simulink model "HostOfSeal"  (R2025a)
settings: Solver=FixedStepDiscrete  StartTime=0.0  StopTime=30  FixedStep=0.025  RelTol=1e-3
model workspace (MATLAB code in the model file + MAT data in the model file):
  | cmdLim = Simulink.Parameter;
  | cmdLim.Value = 15;
  | cmdLim.Description = 'Limit for controlling the maximum surface command angle.';
  | cmdLim.Min = 0;
  | cmdLim.Max = 90;
  | cmdLim.DocUnits = 'deg';
  | 
  | dispGain = Simulink.Parameter;
  | dispGain.Value = 0.75;
  | dispGain.Description = 'Gain applied to the displacement error.';
  | dispGain.Min = 0;
  | dispGain.Max = [];
  | dispGain.DocUnits = 'deg/sec/deg';
  | 
  | dispLim = Simulink.Parameter;
  | dispLim.Value = 30;
  | dispLim.Description = 'Limit for controlling the maximum commanded angle.';
  | dispLim.Min = 0;
  | dispLim.Max = 180;
  | dispLim.DocUnits = 'deg';
  | 
  | intGain = Simulink.Parameter;
  | intGain.Value = 0.5;
  | intGain.Description = 'Gain applied to the integral error.';
  | intGain.Min = 0;
  | intGain.Max = [];
  | intGain.DocUnits = 'deg/sec/deg/sec';
  | 
  | intLim = Simulink.Parameter;
  | intLim.Value = 5;
  | intLim.Description = 'Limit for controlling the maximum commanded angle.';
  | intLim.Min = 0;
  | intLim.Max = 90;
  | intLim.DocUnits = 'deg';
  | 
  | rateGain = Simulink.Parameter;
  | rateGain.Value = 2;
  | rateGain.Description = 'Gain applied to the rate error.';
  | rateGain.Min = 0;
  | rateGain.Max = [];
  | rateGain.DocUnits = 'deg/deg/sec';
  | 
  | rateLim = Simulink.Parameter;
  | rateLim.Value = 6;
  | rateLim.Description = 'Limit for controlling the maximum commanded angle.';
  | rateLim.Min = 0;
  | rateLim.Max = 180;
  | rateLim.DocUnits = 'deg/sec';
  | 
  | hdgGain = Simulink.Parameter;
  | hdgGain.Value = 0.015;
values from neighbouring files (symbols this model uses):
  DriveTs = 100e-6    (= 0.0001)    [simpars.m]
  Jm = 1    [simpars.m]
  KEp = Kt * sqrt(2) / 1.5    [simpars.m]
  Kt = 1    [simpars.m]
  Lm = 1e-3    (= 0.001)    [simpars.m]
  PolePairs = 5    [simpars.m]
  Rm = 1    [simpars.m]
  Vdc = 24    [simpars.m]
undefined symbols (not defined in the file or in its folder): CurrentCommand, DcBusVoltage, EncoderMain, EncoderMainSpeed, Iq, KiSpeed, Kp, KpSpeed, PositionCommand, SpeedCommand, SystemTime
libraries: simulink x1
(part 2 of 2)

== matlab function HostOfSeal/Gft Servo Drive with SEAL/SEAL/100 usec Periodic profiler/MATLAB Function ==
  data: y output double size=[3,1]; G_PosProfilerState data_store_memory; G_PosProfilerData data_store_memory; G_SetupReportBuf data_store_memory
function y  = fcn

global G_PosProfilerState
global G_PosProfilerData
global G_SetupReportBuf

Ts = double( G_PosProfilerData.Ts) ; 
% Copy state for use 

y = zeros(3,1) ; 
if ( G_PosProfilerData.ProfileDataOk == 0 )
    speed =  max( abs(G_PosProfilerState.Speed)-Ts*G_SetupReportBuf.AbsoluteAccelerationLimit , 0 ) * sign(G_PosProfilerState.Speed); 
    pos    = G_PosProfilerState.Position + ( speed + G_PosProfilerState.Speed ) * Ts* 0.5  ;  
    NewFiltState4 = double(pos) ; 
    NewFiltState3 = double(pos) ; 
    NewFiltState2 = double(pos) ; 
    NewFiltState1 = double(pos) ; 
else  
    % Advance profiler 
    Delta = G_PosProfilerData.PositionTarget - G_PosProfilerState.Position - G_PosProfilerState.Speed * Ts * 0.5  ; 
    Direction = 1 ; 
    if ( Delta < 0  )
        Direction = -1 ; 
        Delta = -Delta ;
        speed  = -G_PosProfilerState.Speed ; 
    else
        speed  = G_PosProfilerState.Speed ; 
    end 
        
    desiredSpeed = sqrt(Delta * 2 * G_PosProfilerData.ProfileDeceleration ) ; 
    if ( speed < desiredSpeed  ) 
        speed = min ([speed +Ts * G_PosProfilerData.ProfileDeceleration , G_PosProfilerData.ProfileSpeed  , desiredSpeed] ) ; 
    else
        speed = max(desiredSpeed , speed - Ts * G_PosProfilerData.ProfileDeceleration * 1.02   ) ;  
    end
    speed = speed * Direction ; 

    % tf(2 ,conv([1,2],[1,1.71,1]) )
    pos    = G_PosProfilerState.Position + ( speed +  G_PosProfilerState.Speed ) * Ts* 0.5  ;  
    NewFiltState4 = G_PosProfilerState.FiltState(3) ; 
    NewFiltState3 = G_PosProfilerState.FiltState(2) ; 
    NewFiltState2 = G_PosProfilerState.FiltState(1) ;
    NewFiltState1 = -(G_PosProfilerState.FiltState(1) * G_PosProfilerData.ProfileFilterDen(2) + ...
        G_PosProfilerState.FiltState(2) * G_PosProfilerData.ProfileFilterDen(3) + ...
        G_PosProfilerState.FiltState(3) * G_PosProfilerData.ProfileFilterDen(4)) + double(pos) * G_PosProfilerData.ProfileFilterNum ; 

end
G_PosProfilerState.Position =  double(pos)   ; 
G_PosProfilerState.Speed    =  double(speed) ; 
y = [NewFiltState1 ; (NewFiltState1-G_PosProfilerState.FiltState(1))/ max(Ts,1e-5); 0 ] ;  
G_PosProfilerState.FiltState = [NewFiltState1;NewFiltState2;NewFiltState3;NewFiltState4] ;

end

== matlab function HostOfSeal/Gft Servo Drive with SEAL/SEAL/Idle process UART interpreter/UART message response ==
  data: G_pUartCyclicBuf_in data_store_memory; G_pUartCyclicBuf_out data_store_memory; G_MicroInterp data_store_memory
function UARTHandler()

%global   
global G_MicroInterp      
global G_pUartCyclicBuf_in

for cnt = 1:10 
% The CAN queues count like C (zero based), yet the code here is matlab (1
% based) so we have to increment the counters to be valid Matlab indices
    if (G_pUartCyclicBuf_in.PutCounter == G_pUartCyclicBuf_in.FetchCounter ) 
        return ; 
    end

    nmsgGet     = bitand( G_pUartCyclicBuf_in.FetchCounter, 255) ; 
    nextfetch   = bitand( nmsgGet + 1, 255 ); 
    nextmsg     = G_pUartCyclicBuf_in.UARTQueue(nmsgGet + 1 ) ;
    G_pUartCyclicBuf_in.FetchCounter = nextfetch ; 

    if G_pUartCyclicBuf_in.UartError 
        G_pUartCyclicBuf_in.UartError = uint16(0) ; 
        G_MicroInterp.InterpretError = uint16(3) ; 
        continue ; 
    end

    StringFormatter(nextmsg) ; 
    if ( G_MicroInterp.NewString )
        StringMicroSplitter() ;  
        if G_MicroInterp.InterpretError== uint16(0) 
            MicroInterpret() ; 
            FormatInterpreterResponse() ;
            SendTxResponse();
        end
    end
end
end

function FormatInterpreterResponse() 
    global G_MicroInterp 
    if ( G_MicroInterp.InterpretError) 
        
            
        G_MicroInterp.TempString(1) = 'E' ; 
        G_MicroInterp.TempString(2) = 'R' ; 
        G_MicroInterp.TempString(3) = 'R' ; 
        G_MicroInterp.TempString(4) = 'O' ; 
        G_MicroInterp.TempString(5) = 'R' ; 
        G_MicroInterp.TempString(6) = ':' ; 
        G_MicroInterp.cnt = uint16(6) ; 
        errnum = G_MicroInterp.InterpretError ; 
        while ( errnum )
            G_MicroInterp.cnt = G_MicroInterp.cnt + uint16(1) ;
            nextdigit = uint16(mod( errnum , 10 )) ; 
            G_MicroInterp.TempString(G_MicroInterp.cnt) = nextdigit + uint16('0') ; 
            errnum = errnum - nextdigit ;
        end
    end

    if ( G_MicroInterp.IsGetFunc) 
        n = fix(log10(G_MicroInterp.Argument)) ; 
        SciExp = int16(0) ; 
        SciNotation = 0 ; 
        argout = G_MicroInterp.Argument  ;
        if n > 8 || n < -8   
            nafterPeriod = 8 - n  ; 
        else
            nafterPeriod = 6   ; 
            SciNotation  = 1   ; 
            SciExp = int16(n) ; 
            argout = argout * 10^(-n) ; 
            %n = 1 ; 
        end

        m = fix(argout) ; 
        while ( m )
            G_MicroInterp.cnt = G_MicroInterp.cnt + 1 ;
            nextdigit = uint16(mod( m , 10 )) ; 
            G_MicroInterp.TempString(G_MicroInterp.cnt) = nextdigit + uint16('0') ; 
            m = m - double(nextdigit) ;
        end
        if nafterPeriod > 0 
            G_MicroInterp.cnt = G_MicroInterp.cnt + 1 ;
            G_MicroInterp.TempString(G_MicroInterp.cnt) = '.' ; 
            m = fix( (argout-m) * 10^(nafterPeriod)) ; 
            while ( m )
                G_MicroInterp.cnt = G_MicroInterp.cnt + 1 ;
                nextdigit = uint16(mod( m , 10 )) ; 
                G_MicroInterp.TempString(G_MicroInterp.cnt) = nextdigit + uint16('0') ; 
                m = m - double(nextdigit) ;
            end                
        end
        if SciNotation && SciExp 
            G_MicroInterp.cnt = G_MicroInterp.cnt + 1 ;
            G_MicroInterp.TempString(G_MicroInterp.cnt) = 'E' ; 
            if ( SciExp < 0 )

                G_MicroInterp.cnt = G_MicroInterp.cnt + 1 ;
                G_MicroInterp.TempString(G_MicroInterp.cnt) = '-' ; 
                SciExp = -SciExp ; 
            end
            while ( SciExp )
                G_MicroInterp.cnt = G_MicroInterp.cnt + 1 ;
                nextdigit = uint16(mod( SciExp , 10 )) ; 
                G_MicroInterp.TempString(G_MicroInterp.cnt) = nextdigit + uint16('0') ; 
                SciExp = SciExp - int16(nextdigit) ;
            end                
        end

    end
end


function SendTxResponse()
% Transmit text to a cyclic buffer
    % Return interpreter response 
    global G_pUartCyclicBuf_out  
    global G_MicroInterp      
    for txcnt = 1 : G_MicroInterp.cnt
        nput    = bitand( G_pUartCyclicBuf_out.PutCounter  , 255)  ; 
        nextput = bitand( nput + 1 , 255)  ;  
        if ( nextput == G_pUartCyclicBuf_out.FetchCounter) 
            break ; % Output queue is full 
        end 
        G_pUartCyclicBuf_out.UARTQueue( nput+1) = G_MicroInterp.TempString(txcnt) ; 
    
        % Update TX counter
        G_pUartCyclicBuf_out.PutCounter  = nextput ;
    end
end

function MicroInterpret() 
    global G_MicroInterp      
    switch (G_MicroInterp.MnemonicIndex) 
        case 390 % PA 
            if ( G_MicroInterp.IsGetFunc )
                G_MicroInterp.Argument = GetPositionTarget() ; 
            else
                G_MicroInterp.InterpretError = SetPositionTarget(G_MicroInterp.Argument) ;  
            end
        otherwise
             G_MicroInterp.InterpretError = uint16(22); 

    end
end

function  StringFormatter(c) 

    arguments (Input)
        c uint16 
    end

    global G_MicroInterp      
    
    if ( c == ';' )
        G_MicroInterp.NewString = G_MicroInterp.cnt ; 
        return    ; 
    end
    if G_MicroInterp.NewString 
        G_MicroInterp.cnt = uint16(0) ; 
        G_MicroInterp.InterpretError = uint16(0); 
    end 

    if G_MicroInterp.InterpretError  
        return 
    end

    if ( c <= 'z' && c >= 'a')
        c = c + uint16('A') - uint16('a')   ; 
    end

    if ( c >= 9 && c <= 13) || (c == 32) || (c=='+')
        return ; %  Whitespace - ignore 
    end

    if ( G_MicroInterp.cnt >= 64 )
        G_MicroInterp.InterpretError = uint16(2) ; 
    end

    if ( c <= 'Z' && c >= 'A') || ( c <= '9' && c >= '0') || (c=='-') || (c=='=')
          G_MicroInterp.TempString(G_MicroInterp.cnt+1)  ; 
          G_MicroInterp.cnt = G_MicroInterp.cnt+1 ;
    else
        G_MicroInterp.InterpretError =  uint16(1) ; 
    end

end


function StringMicroSplitter() 
    global G_MicroInterp      
    G_MicroInterp.NewString = uint16(0) ;
    if (G_MicroInterp.cnt < 2 ) 
        return ; 
    end
    if  (G_MicroInterp.TempString(1) < 'A') || (G_MicroInterp.TempString(1) > 'Z') || ...
            (G_MicroInterp.TempString(2) < 'A') || (G_MicroInterp.TempString(2) > 'Z')  
        G_MicroInterp.InterpretError = uint16(10);  
        return ; 
    end
    G_MicroInterp.IsGetFunc  = uint16(1) ; 
    G_MicroInterp.ArrayIndex = uint16(1) ; 
    
    G_MicroInterp.MnemonicIndex = G_MicroInterp.TempString(1) * 26 + G_MicroInterp.TempString(2)  ; 
    
    % Case of scalar GET mnemonic
    if (G_MicroInterp.cnt <= 2 ) 
        return ; 
    end
    
    start = uint16(3) ; 
    if ( G_MicroInterp.TempString(3) =='[')
        gotArrayIndex = uint16(0) ; 
        G_MicroInterp.ArrayIndex = uint16(0) ; 
        for cnt = uint16(4):G_MicroInterp.cnt
            if ( G_MicroInterp.TempString(cnt) == ']')
                if ( G_MicroInterp.ArrayIndex  == 0 ) 
                    G_MicroInterp.InterpretError = uint16(11);  
                    return ; 
                end
                start = cnt + uint16(1) ; 
                gotArrayIndex = uint16(1) ; 
            else
                c = bitand(G_MicroInterp.TempString(cnt), 255 ) ; 
                if ( c < '0' || c > '9')
                    G_MicroInterp.InterpretError =  uint16(12)   ;  
                    return ; 
                end
                G_MicroInterp.ArrayIndex = bitand(G_MicroInterp.ArrayIndex ,31) * 10 + c - uint16('0') ; 
            end
        end
        if ( gotArrayIndex == 0 )
            G_MicroInterp.InterpretError = uint16(14)   ; 
            return ; 
        end
    end

    % Case of vector GET mnemonic
    if (G_MicroInterp.cnt < start ) 
        return ; 
    end
    
    if ~( G_MicroInterp.TempString(start) == '=')
        G_MicroInterp.InterpretError = uint16(15)  ;  
        return ; 
    end
    
    start = start + uint16(1) ;
    Mantissa = 0  ; 
    Exp = uint16(0) ; 
    sgnMant = int16(1) ; 
    sgnExp = int16(1) ; 
    isExp = uint16(0) ; 
    if (G_MicroInterp.cnt < start ) 
        G_MicroInterp.InterpretError = uint16(16)  ;  
        return ; 
    end
    if (G_MicroInterp.TempString(start) == '-')
        sgnMant = int16(-1) ; 
        start = start + uint16(1) ; 
        if (G_MicroInterp.cnt < start ) 
            G_MicroInterp.InterpretError = uint16(17)  ;  
            return ; 
        end
    end

    cnt = start ; 
    WasPeriod = uint16(0); 
    PeriodPos = uint16(0) ; 
    while ( cnt <= G_MicroInterp.cnt) 
        c = bitand(G_MicroInterp.TempString(cnt),255) ;  
        if ( isExp == 0 )
            if ( c >= '0' && c <= '9')
                Mantissa = Mantissa * 10 + double(c)  ; 
                cnt = cnt + uint16(1) ;
                if ( WasPeriod) 
                    PeriodPos = PeriodPos + uint16(1) ;
                end
            else
                if ( c == '.')
                    WasPeriod = uint16(1) ; 
                else
                    if ( c == 'E' )
                        cnt = cnt+ 1 ; 
                        isExp = uint16(1) ;
                        if cnt > G_MicroInterp.cnt
                            G_MicroInterp.InterpretError = uint16(19)  ;  
                            return ; 
                        end
                        if (G_MicroInterp.TempString(cnt) == '-' )
                            sgnExp = int16(-1) ; 
                            cnt = cnt+ uint16(1) ;
                            if cnt > G_MicroInterp.cnt
                                G_MicroInterp.InterpretError = uint16(20)  ;  
                                return ; 
                            end
                        end
                    else
                        G_MicroInterp.InterpretError = uint16(18)  ;  
                        return ; 
                    end
                end
            end
        else
            if ( c >= '0' && c <= '9')
                Exp = bitand(Exp,511) * 10 + c  ; 
                cnt = cnt + 1 ;
            else
                G_MicroInterp.InterpretError = uint16(21)  ;  
                return ;                 
            end
        end
        
    end
    if WasPeriod  
         Mantissa = Mantissa / double(10^single(PeriodPos)) ; 
    end
    G_MicroInterp.Argument = Mantissa * double(sgnMant) ; 
    if isExp
        G_MicroInterp.Argument = G_MicroInterp.Argument * double(10^(single(sgnExp)*single(Exp)) ) ; 
    end

end


function value = GetPositionTarget() 
value = 0 ; 
end

function errcode = SetPositionTarget(pa) 
errcode = uint16(0) ; 
end



% celems(1) = SetBusElement('PutCounter','uint16',"The place in the UARTQueue where the next message is to be put" ) ; 
% celems(2) = SetBusElement('FetchCounter','uint16',"The location in the UARTQueue of the next message to read" ) ; 
% celems(3) = SetBusElement('CANError','uint16',"CAN error" ) ; 
% celems(4) = SetBusElement('UARTQueue','uint32',"Software Queue for incoming UART characters" ,[64,2]) ; 
% celems(5) = SetBusElement('TxFetchCounter','uint16',"The location in the UARTQueue of the next message to transmit" ) ; 
% celems(6) = SetBusElement('CANID','uint32',"Can ID, 11 or 29bit" ,[64,1]) ; 
% celems(7) = SetBusElement('DLenAndAttrib','uint16',"Data length and attributes" ,[64,1]) ;

== matlab function HostOfSeal/Gft Servo Drive with SEAL/SEAL/Drive configuration/MATLAB Function ==
function SealSetup() 

global G_UserInfo

% Object Initialization code 
 SetObject2Drive( uint16(hex2dec('60f0')), uint16(1)  , single(150000) ,VarDataTypes.T_uint32) ; 

% Get object from file 
% G_UserInfo.junk1 = single( GetObjectFromDrive( uint16(hex2dec('60f0')), uint16(1) , VarDataTypes.T_uint32) ) ; 

end


function retCode = SetObject2Drive( Index, subIndex  ,value  , datatype ) 
    retCode = int32(0); 
    coder.ceval('SetObject2Drive', uint16(Index), uint16(subIndex), double(value) , uint16(datatype) ,coder.ref(retCode));
end

function [value,retCode] = GetObjectFromDrive( Index, subIndex , datatype) 
    retCode = int32(0); 
    value   = double(0) ; 
    coder.ceval('GetObjectFromDrive', uint16(Index), uint16(subIndex), uint16(datatype) , coder.ref(value), coder.ref(retCode));
end

== matlab function HostOfSeal/Gft Servo Drive with SEAL/SEAL/Add char to UART/Accept character ==
  data: u input; G_pUartCyclicBuf_in data_store_memory
function ReceiveUartChar(u)

global G_pUartCyclicBuf_in

next = uint16(bitand(G_pUartCyclicBuf_in.PutCounter,255)+ 1) ; 
if ( next == G_pUartCyclicBuf_in.FetchCounter )
    G_pUartCyclicBuf_in.UartError = uint16(1) ; 
    return ; 
end
G_pUartCyclicBuf_in.UARTQueue(G_pUartCyclicBuf_in.PutCounter)  = u ; 
G_pUartCyclicBuf_in.PutCounter = next ;

== matlab function HostOfSeal/Gft Servo Drive with SEAL/SEAL/Copy UART buffer/Get From UART FIFO ==
  data: y output; G_pUartCyclicBuf_out data_store_memory
function y = GetFromUartFifo
global G_pUartCyclicBuf_out 
y = G_pUartCyclicBuf_out ; 
nchars = mod( y.PutCounter - y.FetchCounter, 256 ) ; 
if ( y.PutCounter >= y.FetchCounter)
    y.UARTQueue(1:nchars) = y.UARTQueue(y.FetchCounter:y.FetchCounter+nchars-1) ; 
else
    nrem = 256 - y.FetchCounter + 1  ; 
    y.UARTQueue(1:nrem) = y.UARTQueue(y.FetchCounter:256) ;   
    if ( y.PutCounter > 1 ) 
        y.UARTQueue(nrem+1:nchars)  = y.UARTQueue(1:y.PutCounter-1) ;     
    end
end
y.PutCounter = mod( nchars + 1 , 256) ; 
y.FetchCounter = 1 ; 


% y = uint16([0;0]) ; 
% nchars = mod( G_pUartCyclicBuf_out.PutCounter - G_pUartCyclicBuf_out.FetchCounter, 256 ) ; 
% nextchar = 0 ; 
% if nchars ~= 0 
%     next = uint16(bitand ( G_pUartCyclicBuf_out.FetchCounter, 255) + 1) ; 
%     nextchar = G_pUartCyclicBuf_out.UARTQueue(next) ; 
%     G_pUartCyclicBuf_out.FetchCounter = next ;  
% end
% y(1) = uint16(nextchar) ; 
% y(2) = uint16(nchars) ;

== matlab function HostOfSeal/Gft Servo Drive with SEAL/SEAL/Get CAN Msg to transmit/MATLAB Function ==
  data: y output Bus: CANMessage_T size=1; G_pCANCyclicBuf_out data_store_memory; data input
function y = CanOutTx( data)

global G_pCANCyclicBuf_out 

y = data ; 
if ~(G_pCANCyclicBuf_out.PutCounter == G_pCANCyclicBuf_out.FetchCounter)
    next = uint16(bitand ( G_pCANCyclicBuf_out.FetchCounter, 255) + 1) ; 
    y.CANID = G_pCANCyclicBuf_out.CANID(next) ; 
    y.DataLen = G_pCANCyclicBuf_out.DLenAndAttrib(next) ; 
    y.MsgData(1) =  G_pCANCyclicBuf_out.CANQueue(next*2-1) ; 
    y.MsgData(2) =  G_pCANCyclicBuf_out.CANQueue(next*2) ; 
    y.CANTxCnt = mod( G_pCANCyclicBuf_out.FetchCounter - G_pCANCyclicBuf_out.PutCounter, 64  ) ; 
    G_pCANCyclicBuf_out.FetchCounter = next ;  
end

== matlab function HostOfSeal/Gft Servo Drive with SEAL/SEAL/CanSetRcvMsg/MATLAB Function ==
  data: u input Bus: CANMessage_T size=1; G_pCANCyclicBuf_in data_store_memory
function RcvCanMsg(u)
global G_pCANCyclicBuf_in 

next = bitand(G_pCANCyclicBuf_in.PutCounter, 63) + 1 ; 
if ( next == G_pCANCyclicBuf_in.FetchCounter)
    return ; 
end

G_pCANCyclicBuf_in.CANID(next) = u.CANID ; 
G_pCANCyclicBuf_in.CANQueue(next*2-1:next*2) = u.MsgData(1:2) ; 
G_pCANCyclicBuf_in.DLenAndAttrib(next) = u.DataLen ; 

G_pCANCyclicBuf_in.PutCounter = next ;
